simulink model "b1_cscd_mdl"  (R2020a)
settings: Solver=VariableStepAuto  StartTime=0.0  StopTime=10.0  RelTol=1e-3
settings Model: Creator=soymarwin  LastModifiedBy=soymarwin

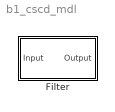
== system b1_cscd_mdl ==
  Filter : Subsystem  Tag=FilterWizardSubSystem
      settings: ErrorFcn=dspFilterRealizedInBasicElemsAlgLoopErrFcnCallback

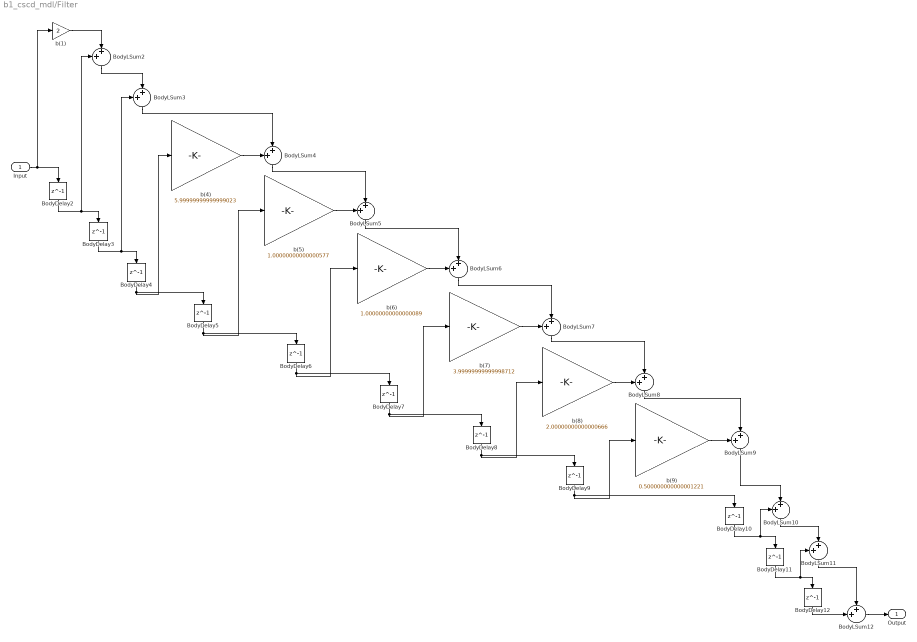
== system b1_cscd_mdl/Filter ==
  Input : Inport
  BodyDelay{2..12} (11 alike) : Delay  DelayLength=1  InitialCondition=0  InputProcessing=Columns as channels (frame based)
  BodyLSum{2..12} (11 alike) : Sum  Inputs=++|  RndMeth=Nearest  SaturateOnIntegerOverflow=on  OutDataTypeStr=Inherit: Same as first input
  b(1) : Gain  Gain=2  ParamDataTypeStr=double  RndMeth=Nearest  SaturateOnIntegerOverflow=on  OutDataTypeStr=Inherit: Same as input
  b(4) : Gain  Gain=5.99999999999999023  ParamDataTypeStr=double  RndMeth=Nearest  SaturateOnIntegerOverflow=on  OutDataTypeStr=Inherit: Same as input
  b(5) : Gain  Gain=1.00000000000000577  ParamDataTypeStr=double  RndMeth=Nearest  SaturateOnIntegerOverflow=on  OutDataTypeStr=Inherit: Same as input
  b(6) : Gain  Gain=1.00000000000000089  ParamDataTypeStr=double  RndMeth=Nearest  SaturateOnIntegerOverflow=on  OutDataTypeStr=Inherit: Same as input
  b(7) : Gain  Gain=3.99999999999998712  ParamDataTypeStr=double  RndMeth=Nearest  SaturateOnIntegerOverflow=on  OutDataTypeStr=Inherit: Same as input
  b(8) : Gain  Gain=2.00000000000000666  ParamDataTypeStr=double  RndMeth=Nearest  SaturateOnIntegerOverflow=on  OutDataTypeStr=Inherit: Same as input
  b(9) : Gain  Gain=0.500000000000001221  ParamDataTypeStr=double  RndMeth=Nearest  SaturateOnIntegerOverflow=on  OutDataTypeStr=Inherit: Same as input
  Output : Outport
  wires:
  BodyLSum12/1 -> Output/1
  BodyLSum9/1 -> BodyLSum10/2
  BodyDelay6/1 -> b(6)/1, BodyDelay7/1
  BodyLSum10/1 -> BodyLSum11/2
  BodyDelay12/1 -> BodyLSum12/2
  b(9)/1 -> BodyLSum9/1
  b(6)/1 -> BodyLSum6/1
  BodyLSum11/1 -> BodyLSum12/1
  BodyLSum8/1 -> BodyLSum9/2
  b(8)/1 -> BodyLSum8/1
  BodyLSum7/1 -> BodyLSum8/2
  b(7)/1 -> BodyLSum7/1
  BodyLSum6/1 -> BodyLSum7/2
  BodyLSum5/1 -> BodyLSum6/2
  b(5)/1 -> BodyLSum5/1
  BodyDelay11/1 -> BodyLSum11/1, BodyDelay12/1
  BodyLSum4/1 -> BodyLSum5/2
  b(4)/1 -> BodyLSum4/1
  BodyDelay4/1 -> b(4)/1, BodyDelay5/1
  BodyLSum3/1 -> BodyLSum4/2
  BodyDelay3/1 -> BodyLSum3/1, BodyDelay4/1
  BodyLSum2/1 -> BodyLSum3/2
  Input/1 -> b(1)/1, BodyDelay2/1
  b(1)/1 -> BodyLSum2/2
  BodyDelay10/1 -> BodyLSum10/1, BodyDelay11/1
  BodyDelay9/1 -> b(9)/1, BodyDelay10/1
  BodyDelay8/1 -> b(8)/1, BodyDelay9/1
  BodyDelay7/1 -> b(7)/1, BodyDelay8/1
  BodyDelay5/1 -> b(5)/1, BodyDelay6/1
  BodyDelay2/1 -> BodyLSum2/1, BodyDelay3/1
